simulink model "HelicopterWithDisturbances"  (R2023b)
settings: Solver=VariableStepAuto  StartTime=0.0  StopTime=20  RelTol=1e-3
InitFcn:
  | % NOTE: If using VoltPAQ-X1, make sure both Gain switches are set to 3.
  | K_AMP = 3;
  | 
  | % Maximum Output Voltage (V): YAW limited to 15 V. PITCH limited to 24 V.
  | VMAX_AMP_P = 24;
  | VMAX_AMP_Y = 15;
  | 
  | % Initial Angle of Pitch (rad)
  | theta_0 = 7*pi/180;
  | phsy_0 = -7*pi/180;
  | 
  | % Performance specifications
  | settle_range_p = 0.003;
  | rise_range_theta_low = 0.1 * theta_0;
  | rise_range_theta_up = 0.9 * theta_0;
  | 
  | rise_range_phsy_low = 0.1 * phsy_0;
  | rise_range_phsy_up = 0.9 * phsy_0;
  | 
  | 
  | g = 9.81;
  | 
  | % Pitch and Yaw Motor Voltage-Torque Constant (N.m/V)
  | % The amount of torque the motor generates per unit of input V   !!
  | K_yp = 0.0219;
  | K_py = 0.0068;
  | 
  | % Pitch and Yaw Viscous Damping Constant (N.m.s/rad)
  | B_p = 0.8;
  | B_y = 0.318;
  | 
  | % Mass of the Helicopter (kg)
  | m = 1.3872;
  | 
  | % Pitch and Yaw Propeller Torque-Thrust Constant found Experimentally (N.m/V)
  | % how much rotational torque is generated by the trust applied on each
  | % motor. Depends on the distance of the point where the trust is applied.
  | % !!
  | K_pp = 0.204;
  | K_yy = 0.072;
  | 
  | % Helicopter Center of Mass from Pivot along Pitch Axis (m)
  | l = 0.186;
  | 
  | J_eq_p = 0.0384;
  | J_eq_y = 0.0432;
  | 
  | A=[      0         0      1.0000                  0
  |          0         0         0                 1.0000
  |          0         0   -B_p/(J_eq_p+m*l^2)        0
  |          0         0         0             -B_y/(J_eq_y+m*l^2)];
  | 
  | B=[      0                     0
  |          0                     0
  |     K_pp/(J_eq_p+m*l^2)   K_py/(J_eq_p+m*l^2)
  |     K_yp/(J_eq_y+m*l^2)   K_yy/(J_eq_y+m*l^2)];
  | 
  | 
  | Q =[35 0 0 0; 0 35 0 0; 0 0 1 0; 0 0 0 1];
  | %Q = eye(4);
  | R = [1 0; 0 1];
  | K = lqr(A,B,Q,R)
  | 
  | u2_star = m*g*l/(K_py - K_pp*K_yy/K_yp);
  | u1_star = -(K_yy * u2_star)/K_yp ;
  | 
  | 
  | % saved gains
  | K_s= [5.87251046470696	0.716673455562105	0.698398143840322	0.167251771048268
  | -0.716673455562108	5.87251046470696	-0.0763535217538760	1.52952706446704]
libraries: dspsrcs4 x2
settings Model: Creator=Sona  LastModifiedBy=Sona

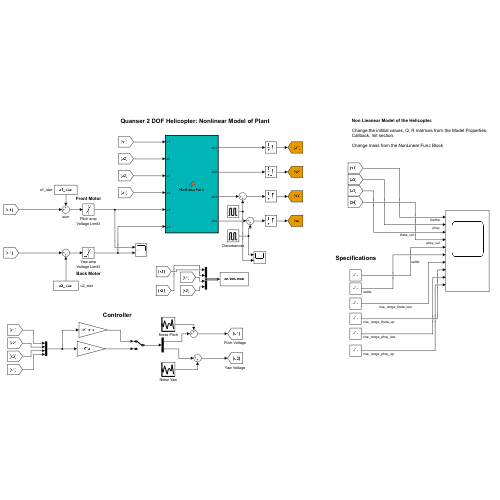
[thumbnail: Simulink's stored preview of the top-level diagram]
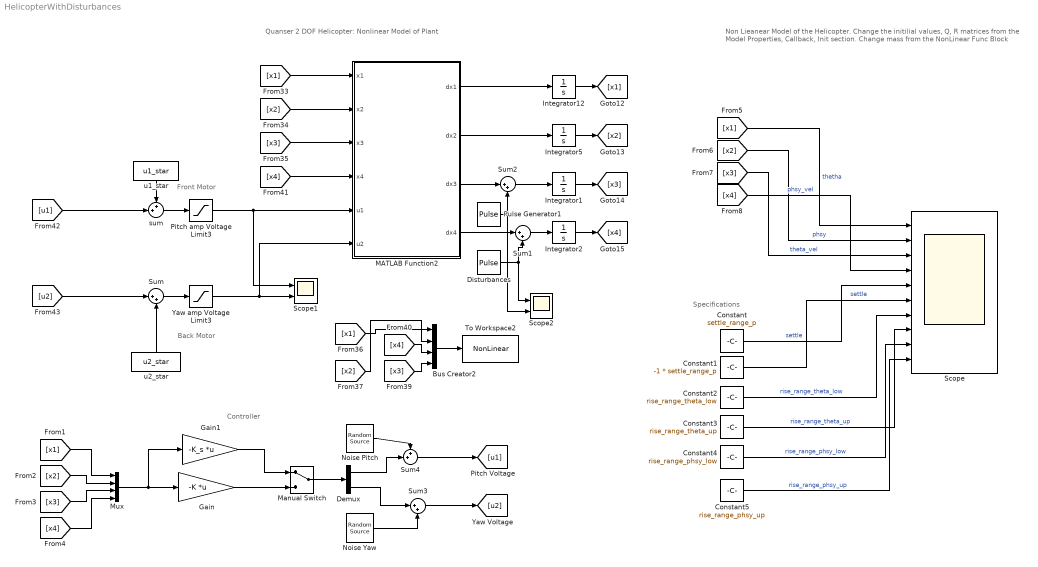
== system HelicopterWithDisturbances ==
  note: Specifications
  note: Non Lieanear Model of the Helicopter.
      |
      | Change the initilial values, Q, R matrices from the Model Properties, Callback, Init section.
      |
      | Change mass from the NonLinear Func Block
  note: Front Motor
  note: Quanser 2 DOF Helicopter: Nonlinear Model of Plant
  note: Controller
  note: Back Motor
  Bus Creator2 : BusCreator  Inputs=4
  Constant : Constant  Value=settle_range_p
  Constant1 : Constant  Value=-1 * settle_range_p
  Constant2 : Constant  Value=rise_range_theta_low
  Constant3 : Constant  Value=rise_range_theta_up
  Constant4 : Constant  Value=rise_range_phsy_low
  Constant5 : Constant  Value=rise_range_phsy_up
  Demux : Demux  Outputs=2
  Disturbances : DiscretePulseGenerator  PulseType=Time based  Amplitude=-0.5  Period=10  PulseWidth=2  PhaseDelay=4
  Gain : Gain  Gain=-K  Multiplication=Matrix(K*u)
  Gain1 : Gain  Gain=-K_s  Multiplication=Matrix(K*u)
  Integrator1 : Integrator  InitialCondition=0.2  LimitOutput=on  UpperSaturationLimit=0.25  LowerSaturationLimit=-0.25
  Integrator12 : Integrator  InitialCondition=theta_0  LimitOutput=on  UpperSaturationLimit=10 * pi/180  LowerSaturationLimit=-10*pi/180
  Integrator2 : Integrator  InitialCondition=-0.2  LimitOutput=on  UpperSaturationLimit=0.25  LowerSaturationLimit=-0.25
  Integrator5 : Integrator  InitialCondition=phsy_0  LimitOutput=on  UpperSaturationLimit=10*pi/180  LowerSaturationLimit=-10*pi/180
  MATLAB Function2 : MATLAB Function  TreatAsAtomicUnit=on
  Manual Switch : ManualSwitch
  Mux : Mux
  Noise Pitch : dspsrcs4/Random Source  SrcType=Gaussian  NormMethod=Ziggurat  CltLength=12  MinVal=0  MaxVal=1  MeanVal=0  VarVal=0.001  RepMode=Not repeatable  rawSeed=1  IsInherit=off  SampMode=Continuous  SampTime=1  SampFrame=1  DataType=Double  OutComplex=Real  OutputFrames=off
  Noise Yaw : dspsrcs4/Random Source  SrcType=Gaussian  NormMethod=Ziggurat  CltLength=12  MinVal=0  MaxVal=1  MeanVal=0  VarVal=0.001  RepMode=Not repeatable  rawSeed=1  IsInherit=off  SampMode=Continuous  SampTime=1  SampFrame=1  DataType=Double  OutComplex=Real  OutputFrames=off
  Pitch amp Voltage Limit3 : Saturate  UpperLimit=VMAX_AMP_P  LowerLimit=- VMAX_AMP_P
  Pulse Generator1 : DiscretePulseGenerator  PulseType=Time based  Amplitude=1.7  Period=10  PulseWidth=2  PhaseDelay=5
  Scope : Scope  NumInputPorts=10
  Scope1 : Scope  NumInputPorts=2
  Scope2 : Scope  NumInputPorts=2
  Sum{,1..3} (4 alike) : Sum  Inputs=|++
  Sum4 : Sum  Inputs=++|
  To Workspace2 : ToWorkspace  VariableName=NonLinear  SampleTime=-1
  Yaw amp Voltage Limit3 : Saturate  UpperLimit=VMAX_AMP_Y  LowerLimit=- VMAX_AMP_Y
  sum : Sum  Inputs=++|
  u1_star : Constant  Value=u1_star
  u2_star : Constant  Value=u2_star
  wires:
  Constant/1 -> Scope/5  "settle"
  [x4] -> Scope/4  "phsy_vel"
  Constant5/1 -> Scope/10  "rise_range_phsy_up"
  Constant2/1 -> Scope/7  "rise_range_theta_low"
  [x1] -> Scope/1  "thetha"
  MATLAB Function2/2(dx2) -> Integrator5/1
  [x2] -> MATLAB Function2/2(x2)
  [x2] -> Scope/2  "phsy"
  Manual Switch/1 -> Demux/1
  Gain/1 -> Manual Switch/2
  [x2] -> Bus Creator2/2
  [x1] -> Bus Creator2/1
  Integrator5/1 -> [x2]
  [x4] -> MATLAB Function2/4(x4)
  Constant4/1 -> Scope/9  "rise_range_phsy_low"
  Integrator12/1 -> [x1]
  [x1] -> Mux/1
  [x4] -> Bus Creator2/3
  Pitch amp Voltage Limit3/1 -> Scope1/1, MATLAB Function2/5(u1)
  [x3] -> Scope/3  "theta_vel"
  Gain1/1 -> Manual Switch/1
  u1_star/1 -> sum/1
  Bus Creator2/1 -> To Workspace2/1
  [x3] -> Mux/3
  Mux/1 -> Gain/1, Gain1/1
  Constant1/1 -> Scope/6  "settle"
  sum/1 -> Pitch amp Voltage Limit3/1
  [x4] -> Mux/4
  Sum/1 -> Yaw amp Voltage Limit3/1
  u2_star/1 -> Sum/2
  [x1] -> MATLAB Function2/1(x1)
  [x2] -> Mux/2
  Integrator1/1 -> [x3]
  [x3] -> MATLAB Function2/3(x3)
  Integrator2/1 -> [x4]
  MATLAB Function2/1(dx1) -> Integrator12/1
  [x3] -> Bus Creator2/4
  Constant3/1 -> Scope/8  "rise_range_theta_up"
  Yaw amp Voltage Limit3/1 -> Scope1/2, MATLAB Function2/6(u2)
  [u2] -> Sum/1
  [u1] -> sum/2
  Sum1/1 -> Integrator2/1
  MATLAB Function2/4(dx4) -> Sum1/1
  MATLAB Function2/3(dx3) -> Sum2/1
  Sum2/1 -> Integrator1/1
  Pulse Generator1/1 -> Scope2/2, Sum2/2
  Sum3/1 -> [u2]
  Demux/2 -> Sum3/1
  Demux/1 -> Sum4/2
  Sum4/1 -> [u1]
  Disturbances/1 -> Sum1/2, Scope2/1
  Noise Pitch/1 -> Sum4/1
  Noise Yaw/1 -> Sum3/2

== matlab function HelicopterWithDisturbances/MATLAB Function2 ==
  data: x1 input; x2 input; x3 input; x4 input; u1 input; dx1 output; u2 input; dx2 output; dx3 output; dx4 output
function [dx1,dx2,dx3,dx4]= NonlinearFunc(x1,x2,x3,x4,u1,u2)
%% Initial Conditions
% Gravitational Constant (m/s^2)
g = 9.81;

% Pitch and Yaw Motor Voltage-Torque Constant (N.m/V)
% The amount of torque the motor generates per unit of input V   !!
K_yp = 0.0219;
K_py = 0.0068;

% Pitch and Yaw Viscous Damping Constant (N.m.s/rad)
B_p = 0.8; 
B_y = 0.318; 

% Mass of the Helicopter (kg)
%m = 1.3872;   % original
m = 1.3773;    % -1%


% Pitch and Yaw Propeller Torque-Thrust Constant found Experimentally (N.m/V)
% how much rotational torque is generated by the trust applied on each
% motor. Depends on the distance of the point where the trust is applied.
% !!
K_pp = 0.204;
K_yy = 0.072;

% Helicopter Center of Mass from Pivot along Pitch Axis (m)
l = 0.186;

J_eq_p = 0.0384;
J_eq_y = 0.0432;
%%
%%

dx1=x3;
dx2=x4;
dx3=(1/(J_eq_p +m*l^2))*((K_pp*u1+K_py*u2)-(B_p*x3+m*l^2*x4^2*sin(x1)*cos(x1)+m*g*l*cos(x1)));
dx4=1/(J_eq_y + m*l^2* (cos(x1))^2 ) * (((K_yp*u1 )+(K_yy*u2 ))-B_y*x4+2*m*l^2*x4*x3*sin(x1)*cos(x1));
